simulink model "untitled"  (R2015a)
settings: Solver=ode45  StartTime=0.0  StopTime=40  RelTol=1e-3
libraries: cstblocks x4
settings Model: Creator=saadc  LastModifiedBy=saadc

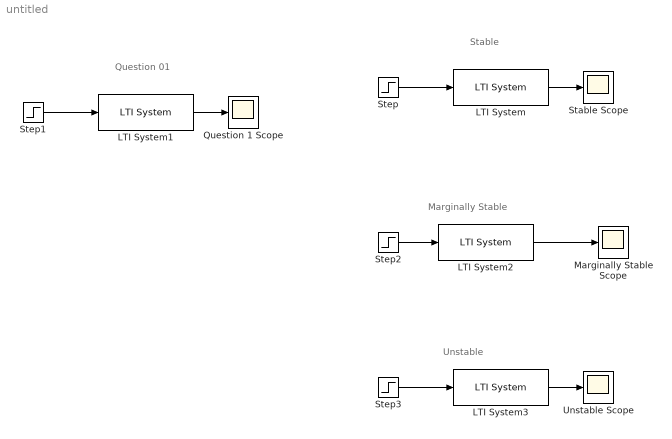
== system untitled ==
  note: Marginally Stable
  note: Stable
  note: Unstable
  note: Question 01
  LTI System : cstblocks/LTI System  sys=tf([5 3],[1 2 17])  IC=[]
  LTI System1 : cstblocks/LTI System  sys=tf(100,[1 4 50])  IC=[]
  LTI System2 : cstblocks/LTI System  sys=tf([4 9],[1 0 4])  IC=[]
  LTI System3 : cstblocks/LTI System  sys=tf([9 4],[1 -6 13])  IC=[]
  Marginally Stable Scope : Scope
      settings: SaveName=ScopeData2
  "Question 1 Scope " : Scope
  Stable Scope : Scope
  Step{,1..3} (4 alike) : Step  SampleTime=0
  "Unstable Scope " : Scope
      settings: SaveName=ScopeData3
  wires:
  Step/1 -> LTI System/1
  LTI System/1 -> Stable Scope/1
  Step2/1 -> LTI System2/1
  LTI System2/1 -> Marginally Stable Scope/1
  Step3/1 -> LTI System3/1
  LTI System3/1 -> "Unstable Scope "/1
  Step1/1 -> LTI System1/1
  LTI System1/1 -> "Question 1 Scope "/1
